simulink model "full_system_LUT"  (R2015b)
settings: Solver=VariableStepAuto  StartTime=0.0  StopTime=10  RelTol=1e-3
values from neighbouring files (symbols this model uses):
  c_drag = -1/2*1.3*.804*.6    (= -0.31356)    [Parameters.m]
  G1 = 12    [Parameters.m]
  G2 = 50    [Parameters.m]
  J_G1 = (.01*G1/(2*pi)).^4*pi*8050*.01/2    [Parameters.m]
  J_M = 52e-4    (= 0.0052)    [Parameters.m]
  Kt = .07329    (= 0.07329)    [Parameters.m]
  L = 1e-4/2    (= 5e-05)    [Parameters.m]
  N = 4    [Parameters.m]
  phase_3 = -1/6*cos(3*(x+pi/2))    [Parameters.m]
  phase_a = cos(x+pi/2)    [Parameters.m]
  phase_b = cos(x+pi/2-2*pi/3)    [Parameters.m]
  phase_c = cos(x+pi/2+2*pi/3)    [Parameters.m]
  r = 11*.0254/2    (= 0.1397)    [Parameters.m]
  x = Input_range(1):(1/Encoder_res):Input_range(2)    [Parameters.m]
undefined symbols (not defined in the file or in its folder): sigbuilder_block
libraries: fl_lib x25, nesl_utility x12, pe_lib x3
settings Model: Creator=Martin Andersen  LastModifiedBy=Martin Andersen

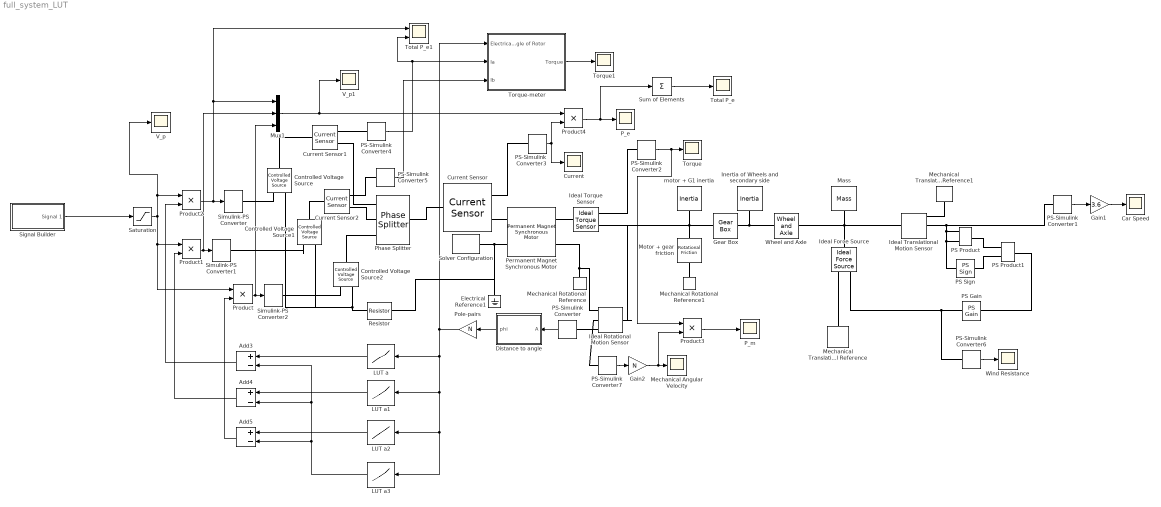
== system full_system_LUT ==
  Add3 : Sum  Inputs=+-
  Add4 : Sum  Inputs=+-
  Add5 : Sum  Inputs=+-
  Car Speed : Scope
  Controlled Voltage Source : fl_lib/Electrical/Electrical Sources/Controlled Voltage Source
  Controlled Voltage Source1 : fl_lib/Electrical/Electrical Sources/Controlled Voltage Source
  Controlled Voltage Source2 : fl_lib/Electrical/Electrical Sources/Controlled Voltage Source
  Current : Scope
  Current Sensor : pe_lib/Sensors/Current Sensor
  Current Sensor1 : fl_lib/Electrical/Electrical Sensors/Current Sensor
  Current Sensor2 : fl_lib/Electrical/Electrical Sensors/Current Sensor
  Distance to angle : MATLAB Function  TreatAsAtomicUnit=on
  Electrical Reference1 : fl_lib/Electrical/Electrical Elements/Electrical Reference
  Gain1 : Gain  Gain=3.6
  Gain2 : Gain  Gain=N
  Gear Box : fl_lib/Mechanical/Mechanisms/Gear Box  ratio=G2/G1  t_in_specify=off  t_in_priority=None  t_in=0 N*m  t_out_specify=off  t_out_priority=None  t_out=0 N*m
  Ideal Force Source : fl_lib/Mechanical/Mechanical Sources/Ideal Force Source
  Ideal Rotational Motion Sensor : fl_lib/Mechanical/Mechanical Sensors/Ideal Rotational Motion Sensor  offset=0 rad
  Ideal Torque Sensor : fl_lib/Mechanical/Mechanical Sensors/Ideal Torque Sensor
  Ideal Translational Motion Sensor : fl_lib/Mechanical/Mechanical Sensors/Ideal Translational Motion Sensor  offset=0 m
  Inertia of Wheels and secondary side : fl_lib/Mechanical/Rotational Elements/Inertia  inertia=J_M + J_G1 kg*m^2  w_specify=off  w_priority=None  w=0 rad/s  t_specify=off  t_priority=None  t=0 N*m
  LUT a : Lookup_n-D  NumberOfTableDimensions=1  BreakpointsForDimension1=x  BeginIndexSearchUsingPreviousIndexResult=on  Table=phase_a  InterpMethod=Flat  InternalRulePriority=Speed  RndMeth=Simplest  InputSameDT=on
  LUT a1 : Lookup_n-D  NumberOfTableDimensions=1  BreakpointsForDimension1=x  BeginIndexSearchUsingPreviousIndexResult=on  Table=phase_b  InterpMethod=Flat  InternalRulePriority=Speed  RndMeth=Simplest  InputSameDT=on
  LUT a2 : Lookup_n-D  NumberOfTableDimensions=1  BreakpointsForDimension1=x  BeginIndexSearchUsingPreviousIndexResult=on  Table=phase_c  InterpMethod=Flat  InternalRulePriority=Speed  RndMeth=Simplest  InputSameDT=on
  LUT a3 : Lookup_n-D  NumberOfTableDimensions=1  BreakpointsForDimension1=x  BeginIndexSearchUsingPreviousIndexResult=on  Table=phase_3  InterpMethod=Flat  InternalRulePriority=Speed  RndMeth=Simplest  InputSameDT=on
  Mass : fl_lib/Mechanical/Translational Elements/Mass  mass=m kg  v_specify=off  v_priority=None  v=0 m/s  f_specify=off  f_priority=None  f=0 N
  Mechanical Angular Velocity : Scope
  Mechanical Rotational Reference : fl_lib/Mechanical/Rotational Elements/Mechanical Rotational Reference
  Mechanical Rotational Reference1 : fl_lib/Mechanical/Rotational Elements/Mechanical Rotational Reference
  Mechanical Translational Reference : fl_lib/Mechanical/Translational Elements/Mechanical Translational Reference
  Mechanical Translational Reference1 : fl_lib/Mechanical/Translational Elements/Mechanical Translational Reference
  Motor + gear friction : fl_lib/Mechanical/Rotational Elements/Rotational Friction  brkwy_trq=.5 N*m  Col_trq=.2 N*m  visc_coef=0.0001 N*m/(rad/s)  trans_coef=10 s/rad  vel_thr=1e-4 rad/s  w_specify=off  w_priority=None  w=0 rad/s  t_specify=off  t_priority=None  t=0 N*m
  Mux1 : Mux  Inputs=3
  PS Gain : fl_lib/Physical Signals/Functions/PS Gain  gain=c_drag
  PS Product : fl_lib/Physical Signals/Functions/PS Product
  PS Product1 : fl_lib/Physical Signals/Functions/PS Product
  PS Sign : fl_lib/Physical Signals/Nonlinear Operators/PS Sign
  PS-Simulink Converter{,1..7} (8 alike) : nesl_utility/PS-Simulink Converter  PhysicalDomain=network_engine_domain  SubClassName=ps_output  LeftPortType=input  RightPortType=output  PseudoPeriodic=off  Frequencies=[]  Unit=1  AffineConversion=off
  P_e : Scope
  P_m : Scope
  Permanent Magnet Synchronous Motor : pe_lib/Machines/Permanent Magnet Rotor/Permanent Magnet Synchronous Motor  nPolePairs=N  pm_flux_linkage=Kt/N Wb  stator_param=2  Ld=.1 mH  Lq=.1 mH  L0=.1 mH  Ls=L H  Lm=0 H  Ms=L/10 H  Rs=R Ohm  initial_currents=[0, 0, 0] A  axes_param=2  angular_position0=0 rad  rotor_offset=- pi / 2 rad  shift_3ph=[nan, nan, nan] rad  sqrt2OverSqrt3=nan  oneOverSqrt2=nan  twoPiOver3=nan  Lmin=1e-9 H
  Phase Splitter : pe_lib/Connections/Phase Splitter
  Pole-pairs : Gain  Gain=N
  Product{,1..4} (5 alike) : Product
  Resistor : fl_lib/Electrical/Electrical Elements/Resistor  R=1e9 Ohm  i_specify=off  i_priority=None  i=0 A  v_specify=off  v_priority=None  v=0 V
  Saturation : Saturate  UpperLimit=26*2/sqrt(3)  LowerLimit=-26*2/sqrt(3)
  Signal Builder : Subsystem  Tag=STV Subsys  LoadFcn=sigbuilder_block('load');  StartFcn=sigbuilder_block('start');  StopFcn=sigbuilder_block('stop');  ClipboardFcn=sigbuilder_block('clipboard');  mask(Sigbuilder block){}
      mask help: Simulink:masks:SigbuilderBlock_MD
      mask init:
      | if ~strcmp(get_param(bdroot(gcbh),'SimulationStatus'),'stopped') tuvar = sigbuilder_block('maskInit'); end
      settings: CopyFcn=sigbuilder_block('copy');  DeleteFcn=sigbuilder_block('delete');  ModelCloseFcn=sigbuilder_block('modelClose');  PreSaveFcn=sigbuilder_block('preSave');  PauseFcn=sigbuilder_block('pause');  ContinueFcn=sigbuilder_block('continue');  NameChangeFcn=sigbuilder_block('namechange');  OpenFcn=sigbuilder_block('open',[409.8 160.8 550.8 400.2 ]);  CloseFcn=sigbuilder_block('close');
      mask Display: plot(0, 0, 100, 100,[2, 2, 32, 32, 2], [68, 8, 8, 68, 68],[32, 2], [38, 38], [32, 19, 2],[53, 60, 44], [32, 17, 17, 2],[16, 16, 31, 31]);txt = getActiveGroup(gcbh);text(2, 100, txt,'verticalAlignment', 'top');
  Simulink-PS Converter : nesl_utility/Simulink-PS Converter  PhysicalDomain=network_engine_domain  SubClassName=ps_input  LeftPortType=input  RightPortType=output  PseudoPeriodic=off  Frequencies=[]  NoiseDistribution=none  NoiseParameters=[]  Unit=1  AffineConversion=off  InputFiltering=off  SimscapeFilterOrder=1  InputFilterTimeConstant=0.001  UdotUserProvided=1
  Simulink-PS Converter1 : nesl_utility/Simulink-PS Converter  PhysicalDomain=network_engine_domain  SubClassName=ps_input  LeftPortType=input  RightPortType=output  PseudoPeriodic=off  Frequencies=[]  NoiseDistribution=none  NoiseParameters=[]  Unit=1  AffineConversion=off  InputFiltering=off  SimscapeFilterOrder=1  InputFilterTimeConstant=0.001  UdotUserProvided=1
  Simulink-PS Converter2 : nesl_utility/Simulink-PS Converter  PhysicalDomain=network_engine_domain  SubClassName=ps_input  LeftPortType=input  RightPortType=output  PseudoPeriodic=off  Frequencies=[]  NoiseDistribution=none  NoiseParameters=[]  Unit=1  AffineConversion=off  InputFiltering=off  SimscapeFilterOrder=1  InputFilterTimeConstant=0.001  UdotUserProvided=1
  Solver Configuration : nesl_utility/Solver Configuration  PhysicalDomain=network_engine_domain  SubClassName=solver  LeftPortType=input  RightPortType=generic  Accelerate=off  Tones=[]  Harmonics=[]  SimulateNoise=off  Profile=off  UseLocalSampling=off  EnableSwitchedLinearOptims=on  FrequencyDomain=off  UseCCode=off  RelTol=0.001  AbsTol=1e-06  MinStep=1e-09  ToWorkspace=off  RevertToSquareIcSolve=off  NumHomotopyIterations=100  PhasorMode=off  PhasorModeNumHarmonics=1  DoDC=off  ResidualTolerance=1e-09  UseLocalSolver=off  LocalSolverChoice=NE_BACKWARD_EULER_ADVANCER  LocalSolverSampleTime=0.001  DoFixedCost=off  MaxNonlinIter=3  MaxModeIter=2  LinearAlgebra=Sparse  DelaysMemoryBudget=1024  AutomaticFiltering=on  FilteringTimeConstant=0.001
  Sum of Elements : Sum  Inputs=+
  Torque : Scope
  Torque-meter : Subsystem
  Torque1 : Scope
  Total P_e : Scope
  Total P_e1 : Scope  NumInputPorts=2
  V_p : Scope
  V_p1 : Scope
  Wheel and Axle : fl_lib/Mechanical/Mechanisms/Wheel and Axle  R=r m  or=1  orient=1  t_specify=off  t_priority=None  t=0 N*m  f_specify=off  f_priority=None  f=0 N
  Wind Resistance : Scope
  motor + G1 inertia : fl_lib/Mechanical/Rotational Elements/Inertia  inertia=J_M + J_G1 kg*m^2  w_specify=off  w_priority=None  w=0 rad/s  t_specify=off  t_priority=None  t=0 N*m
  wires:
  Product2/1 -> Total P_e1/1, Mux1/1, Simulink-PS Converter/1
  Product1/1 -> Mux1/2, Simulink-PS Converter1/1
  Product/1 -> Mux1/3, Simulink-PS Converter2/1
  PS-Simulink Converter/1 -> Distance to angle/1(A)
  PS-Simulink Converter3/1 -> Product4/2, Current/1
  PS-Simulink Converter1/1 -> Gain1/1
  Gain1/1 -> Car Speed/1
  PS-Simulink Converter2/1 -> Product3/1, Torque/1
  PS-Simulink Converter4/1 -> Torque-meter/2(Ia), Total P_e1/2
  PS-Simulink Converter5/1 -> Torque-meter/3(Ib)
  Pole-pairs/1 -> LUT a3/1, LUT a2/1, LUT a1/1, LUT a/1, Torque-meter/1(Electrical Angle of Rotor)
  Signal Builder/1(Signal 1) -> Saturation/1
  Saturation/1 -> V_p/1, Product2/1, Product/1, Product1/1
  Torque-meter/1(Torque) -> Torque1/1
  PS-Simulink Converter6/1 -> Wind Resistance/1
  PS-Simulink Converter7/1 -> Gain2/1
  Gain2/1 -> Product3/2, Mechanical Angular Velocity/1
  Product3/1 -> P_m/1
  Mux1/1 -> V_p1/1, Product4/1
  Product4/1 -> Sum of Elements/1, P_e/1
  Sum of Elements/1 -> Total P_e/1
  Add5/1 -> Product/2
  Add3/1 -> Product2/2
  Add4/1 -> Product1/2
  LUT a/1 -> Add3/1
  LUT a1/1 -> Add4/1
  LUT a2/1 -> Add5/1
  LUT a3/1 -> Add5/2, Add4/2, Add3/2
  Distance to angle/1(phi) -> Pole-pairs/1
  connections:
  Permanent Magnet Synchronous Motor/LConn2 -- Resistor/RConn1 -- Electrical Reference1/LConn1 -- Solver Configuration/RConn1
  Mechanical Rotational Reference/LConn1 -- Ideal Rotational Motion Sensor/RConn1 -- Permanent Magnet Synchronous Motor/RConn2
  motor + G1 inertia/LConn1 -- Ideal Rotational Motion Sensor/LConn1 -- Ideal Torque Sensor/RConn1 -- Motor + gear friction/LConn1 -- Gear Box/LConn1
  Inertia of Wheels and secondary side/LConn1 -- Gear Box/RConn1 -- Wheel and Axle/LConn1
  Mass/LConn1 -- Ideal Force Source/LConn1 -- Ideal Translational Motion Sensor/LConn1 -- Wheel and Axle/RConn1
  Mechanical Translational Reference/LConn1 -- Ideal Force Source/RConn2
  Mechanical Translational Reference1/LConn1 -- Ideal Translational Motion Sensor/RConn1
  PS Sign/LConn1 -- PS Product/LConn1 -- PS-Simulink Converter1/LConn1 -- Ideal Translational Motion Sensor/RConn2 -- PS Product/LConn2
  PS Product1/LConn2 -- PS Sign/RConn1
  PS Product1/LConn1 -- PS Product/RConn1
  PS Gain/LConn1 -- PS Product1/RConn1
  PS Gain/RConn1 -- PS-Simulink Converter6/LConn1 -- Ideal Force Source/RConn1
  PS-Simulink Converter/LConn1 -- Ideal Rotational Motion Sensor/RConn3
  Controlled Voltage Source/RConn1 -- Simulink-PS Converter/RConn1
  Controlled Voltage Source1/RConn1 -- Simulink-PS Converter1/RConn1
  Controlled Voltage Source2/RConn1 -- Simulink-PS Converter2/RConn1
  Controlled Voltage Source2/LConn1 -- Phase Splitter/RConn3
  Controlled Voltage Source1/RConn2 -- Controlled Voltage Source/RConn2 -- Controlled Voltage Source2/RConn2 -- Resistor/LConn1
  Current Sensor/LConn1 -- Phase Splitter/LConn1
  Permanent Magnet Synchronous Motor/LConn1 -- Current Sensor/RConn2
  PS-Simulink Converter3/LConn1 -- Current Sensor/RConn1
  Ideal Torque Sensor/LConn1 -- Permanent Magnet Synchronous Motor/RConn1
  PS-Simulink Converter2/LConn1 -- Ideal Torque Sensor/RConn2
  Current Sensor1/LConn1 -- Controlled Voltage Source/LConn1
  Current Sensor1/RConn2 -- Phase Splitter/RConn1
  Current Sensor2/LConn1 -- Controlled Voltage Source1/LConn1
  Current Sensor2/RConn2 -- Phase Splitter/RConn2
  PS-Simulink Converter4/LConn1 -- Current Sensor1/RConn1
  Current Sensor2/RConn1 -- PS-Simulink Converter5/LConn1
  Mechanical Rotational Reference1/LConn1 -- Motor + gear friction/RConn1
  PS-Simulink Converter7/LConn1 -- Ideal Rotational Motion Sensor/RConn2

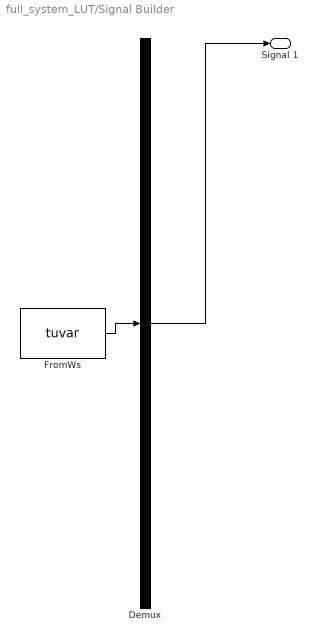
== system full_system_LUT/Signal Builder ==
  Demux : Demux  Tag=STV Demux  Outputs=1
  FromWs : FromWorkspace  Tag=STV FromWs  VariableName=tuvar  SampleTime=0
      SigBuilderData=|
      | common.afterFinalStr = 'Extrapolate'
      | common.sampleTime = 0
      | dataSet.timeRange = [0 30]
      | dataSet.name = 'Group 1'
      | sbobj.Groups.Name = 'Group 1'
      | sbobj.Groups.Signals.Name = 'Signal 1'
      | sbobj.Groups.Signals.XData = [0 0.3 1.05 5.15 10 20 20 30]
      | sbobj.Groups.Signals.YData = [30.2 28.8 29.2 30 30 12.2 12 12]
      | sbobj.Groups.TimeRange = [0 30]
  Signal 1 : Outport  Tag=STV Outport
  wires:
  Demux/1 -> Signal 1/1
  FromWs/1 -> Demux/1

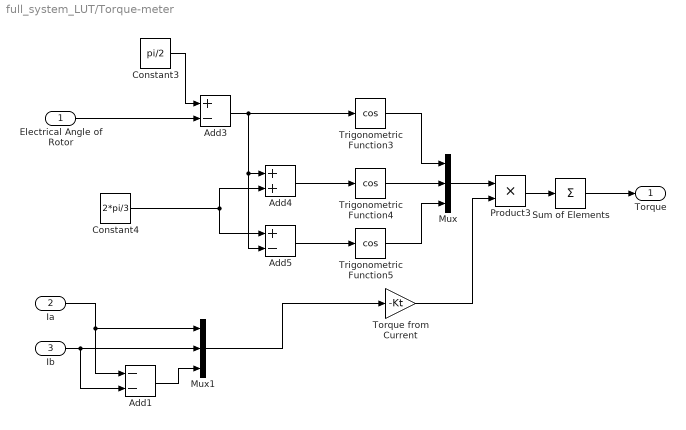
== system full_system_LUT/Torque-meter ==
  Electrical Angle of Rotor : Inport
  Ia : Inport  Port=2
  Ib : Inport  Port=3
  Add1 : Sum  Inputs=--
  Add3 : Sum  Inputs=+-
  Add4 : Sum
  Add5 : Sum  Inputs=+-
  Constant3 : Constant  Value=pi/2
  Constant4 : Constant  Value=2*pi/3
  Mux : Mux  Inputs=3
  Mux1 : Mux  Inputs=3
  Product3 : Product
  Sum of Elements : Sum  Inputs=+
  Torque from Current : Gain  Gain=-Kt
  Trigonometric Function3 : Trigonometry  Operator=cos
  Trigonometric Function4 : Trigonometry  Operator=cos
  Trigonometric Function5 : Trigonometry  Operator=cos
  Torque : Outport
  wires:
  Add4/1 -> Trigonometric Function4/1
  Constant4/1 -> Add4/2, Add5/1
  Trigonometric Function5/1 -> Mux/3
  Mux/1 -> Product3/1
  Torque from Current/1 -> Product3/2
  Constant3/1 -> Add3/1
  Trigonometric Function4/1 -> Mux/2
  Product3/1 -> Sum of Elements/1
  Add5/1 -> Trigonometric Function5/1
  Trigonometric Function3/1 -> Mux/1
  Add3/1 -> Trigonometric Function3/1, Add5/2, Add4/1
  Sum of Elements/1 -> Torque/1
  Electrical Angle of Rotor/1 -> Add3/2
  Ia/1 -> Mux1/1, Add1/1
  Ib/1 -> Mux1/2, Add1/2
  Add1/1 -> Mux1/3
  Mux1/1 -> Torque from Current/1

== matlab function full_system_LUT/Distance to angle ==
  data: A input; phi output
function phi = winddown(A)
persistent c;
if isempty(c)
    c=0;
end
a=A+c*pi*2;
if a > pi
    c=c-1;
    a=A+c*pi*2;
elseif a < -pi
    c=c+1;
    a=A+c*pi*2;
end

phi = a;
end
